simulink model "MICROBOT_1"  (R2015a)
settings: Solver=ode3  StartTime=0.0  StopTime=inf  FixedStep=0.001  RelTol=1e-3
values from neighbouring files (symbols this model uses):
  s = serial('COM4','BaudRate',9600,'DataBits', 8,'Terminator',13)    [start.m]
libraries: mblibv1 x39
settings Model: Creator=anhkh  LastModifiedBy=anhkh
settings SimMechanicsCC: VisOnUpdateDiagram=on  VisDuringSimulation=on

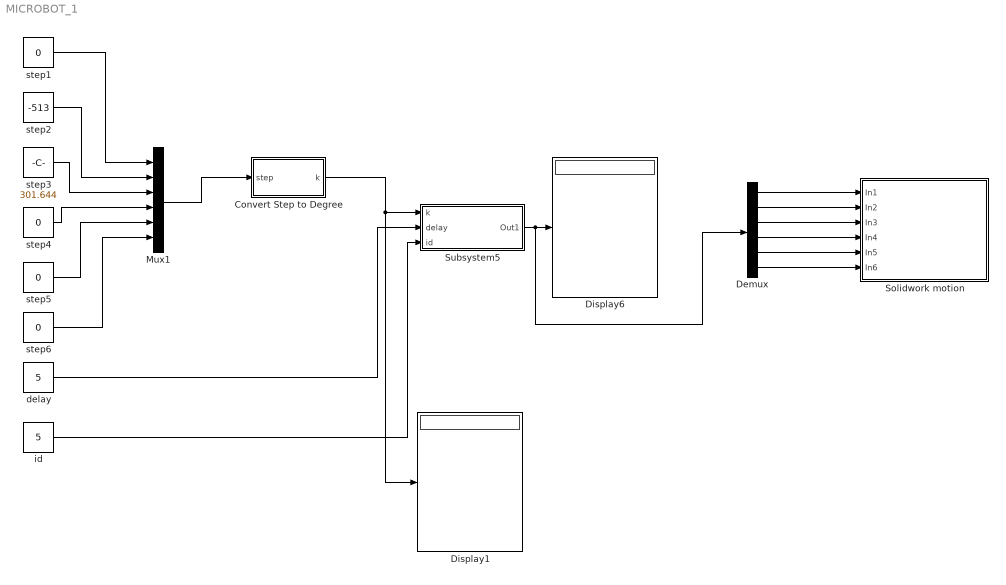
== system MICROBOT_1 ==
  Convert Step to Degree : MATLAB Function  TreatAsAtomicUnit=on
  Demux : Demux  Outputs=6
  Display1 : Display
  Display6 : Display
  Mux1 : Mux  Inputs=6
  Solidwork motion : Subsystem
  Subsystem5 : Subsystem
  delay : Constant  Value=5
  id : Constant  Value=5
  step{1,4..6} (4 alike) : Constant  Value=0
  step2 : Constant  Value=-513
  step3 : Constant  Value=301.644
  wires:
  delay/1 -> Subsystem5/2(delay)
  id/1 -> Subsystem5/3(id)
  Demux/1 -> Solidwork motion/1(In1)
  Demux/2 -> Solidwork motion/2(In2)
  Demux/3 -> Solidwork motion/3(In3)
  Demux/4 -> Solidwork motion/4(In4)
  Demux/5 -> Solidwork motion/5(In5)
  Demux/6 -> Solidwork motion/6(In6)
  Subsystem5/1(Out1) -> Demux/1, Display6/1
  Mux1/1 -> Convert Step to Degree/1(step)
  Convert Step to Degree/1(k) -> Display1/1, Subsystem5/1(k)
  step1/1 -> Mux1/1
  step2/1 -> Mux1/2
  step3/1 -> Mux1/3
  step4/1 -> Mux1/4
  step5/1 -> Mux1/5
  step6/1 -> Mux1/6

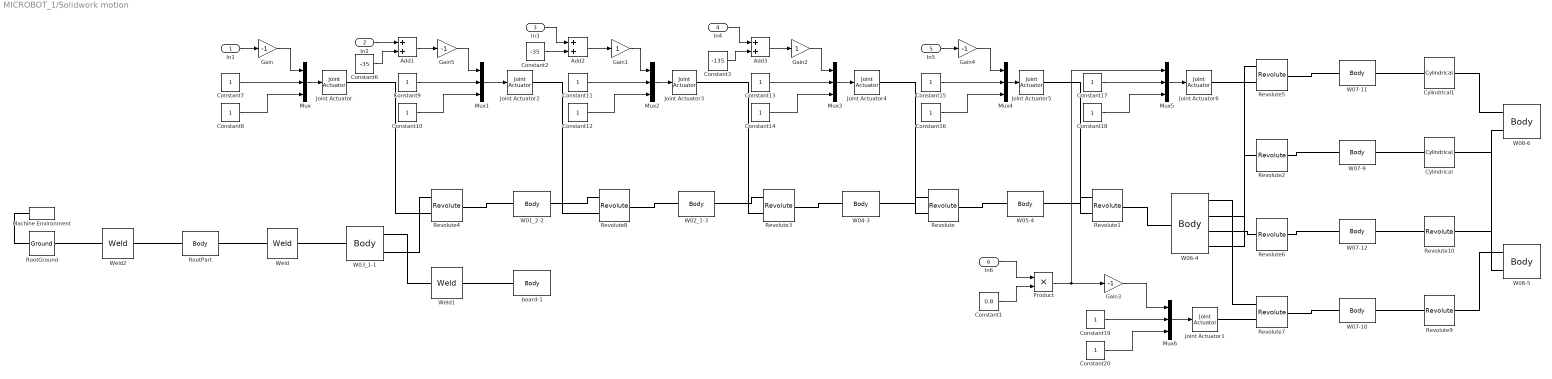
== system MICROBOT_1/Solidwork motion ==
  In1 : Inport
  In2 : Inport  Port=2
  In3 : Inport  Port=3
  In4 : Inport  Port=4
  In5 : Inport  Port=5
  In6 : Inport  Port=6
  Add1 : Sum
  Add2 : Sum
  Add3 : Sum
  Constant1 : Constant  Value=0.8
  Constant{7..20} (14 alike) : Constant
  Constant2 : Constant  Value=-35
  Constant3 : Constant  Value=-135
  Constant6 : Constant  Value=-35
  Cylindrical : mblibv1/Joints/Cylindrical  LConnTagsString=__newl0  RConnTagsString=__newr0  UpdateFromCAD=on  NumSAPorts=0  CutJoint=off  MarkAsCut=off  Primitives=prismatic  PrimitiveProps=P1$WORLD$[0.906308,0,-0.422618]$prismatic#R1$WORLD$[0.906308,0,-0.422618]$revolute  DialogClass=JointBlock  P1Axis=[0.906308,0,-0.422618]  R1Axis=[0.906308,0,-0.422618]
  Cylindrical1 : mblibv1/Joints/Cylindrical  LConnTagsString=__newl0  RConnTagsString=__newr0  UpdateFromCAD=on  NumSAPorts=0  CutJoint=off  MarkAsCut=off  Primitives=prismatic  PrimitiveProps=P1$WORLD$[-0.906308,0,0.422618]$prismatic#R1$WORLD$[0.906308,0,-0.422618]$revolute  DialogClass=JointBlock  P1Axis=[-0.906308,0,0.422618]  R1Axis=[0.906308,0,-0.422618]
  Gain{,3..5} (4 alike) : Gain  Gain=-1
  Gain1 : Gain
  Gain2 : Gain
  Joint Actuator{,1..6} (7 alike) : mblibv1/Sensors &  Actuators/Joint Actuator  UpdateFromCAD=off  PhysicalDomain=Mechanical  PortType=blob  ActuationStyle=Motion  AngleUnits=deg  ArcVelocityUnits=deg/s  ArcAccelerationUnits=deg/s^2  CoordPositionUnits=m  VelocityUnits=m/s  AccelerationUnits=m/s^2  ForceUnits=N  TorqueUnits=N*m  ActiveIO=on  Width=3  DialogClass=MechanicalActuatorBlock  Primitive=R1  ReferenceFrame=Absolute (World)
  Machine Environment : mblibv1/Bodies/Machine Environment  PortType=env  PhysicalDomain=Mechanical  DialogTemplateClass=MECH.MachineEnvironment  SyncWhenCopied=off  Gravity=[0 -9.81 0]  GravityUnits=m/s^2  GravityAsSignal=off  Dimensionality=Auto-detect  AnalysisType=Forward dynamics  LinearAssemblyTolerance=1e-3  LinearAssemblyToleranceUnits=m  AngularAssemblyTolerance=1e-3  AngularAssemblyToleranceUnits=rad  ConstraintSolverType=Stabilizing  ConstraintRelTolerance=1e-4  ConstraintAbsTolerance=1e-4  UseRobustSingularityHandling=off  RedundancyAnalysisToleranceType=Automatically select tolerance  RedundancyAnalysisTolerance=1e-14  StatePerturbationType=Fixed  PerturbationSize=1e-5  VisualizeMachine=on  BodyVisualizationType=Use model default body geometries  BodyColorSelMode=Use model default  DefaultBodyColor=[1 0 0]
  Mux{,1..6} (7 alike) : Mux  Inputs=3
  Product : Product
  Revolute : mblibv1/Joints/Revolute  LConnTagsString=__newl0|SA1  RConnTagsString=__newr0  UpdateFromCAD=on  NumSAPorts=1  CutJoint=off  MarkAsCut=off  Primitives=prismatic  PrimitiveProps=R1$WORLD$[0,1,0]$revolute  DialogClass=JointBlock  R1Axis=[0,1,0]
  Revolute1 : mblibv1/Joints/Revolute  LConnTagsString=__newl0|SA1  RConnTagsString=__newr0  UpdateFromCAD=on  NumSAPorts=1  CutJoint=off  MarkAsCut=off  Primitives=prismatic  PrimitiveProps=R1$WORLD$[0.422618,0,0.906308]$revolute  DialogClass=JointBlock  R1Axis=[0.422618,0,0.906308]
  Revolute10 : mblibv1/Joints/Revolute  LConnTagsString=__newl0  RConnTagsString=__newr0  UpdateFromCAD=on  NumSAPorts=0  CutJoint=off  MarkAsCut=off  Primitives=prismatic  PrimitiveProps=R1$WORLD$[0.906308,0,-0.422618]$revolute  DialogClass=JointBlock  R1Axis=[0.906308,0,-0.422618]
  Revolute2 : mblibv1/Joints/Revolute  LConnTagsString=__newl0  RConnTagsString=__newr0  UpdateFromCAD=on  NumSAPorts=0  CutJoint=off  MarkAsCut=off  Primitives=prismatic  PrimitiveProps=R1$World$[-0.906308,0,0.422618]$revolute  DialogClass=JointBlock  R1Axis=[-0.906308,0,0.422618]
  Revolute3 : mblibv1/Joints/Revolute  LConnTagsString=__newl0|SA1  RConnTagsString=__newr0  UpdateFromCAD=on  NumSAPorts=1  CutJoint=off  MarkAsCut=off  Primitives=prismatic  PrimitiveProps=R1$WORLD$[0,1,0]$revolute  DialogClass=JointBlock  R1Axis=[0,1,0]
  Revolute4 : mblibv1/Joints/Revolute  LConnTagsString=__newl0|SA1  RConnTagsString=__newr0  UpdateFromCAD=on  NumSAPorts=1  CutJoint=off  MarkAsCut=off  Primitives=prismatic  PrimitiveProps=R1$WORLD$[0,0,-1]$revolute  DialogClass=JointBlock  R1Axis=[0,0,-1]
  Revolute5 : mblibv1/Joints/Revolute  LConnTagsString=__newl0|SA1  RConnTagsString=__newr0  UpdateFromCAD=on  NumSAPorts=1  CutJoint=off  MarkAsCut=off  Primitives=prismatic  PrimitiveProps=R1$WORLD$[-0.906308,0,0.422618]$revolute  DialogClass=JointBlock  R1Axis=[-0.906308,0,0.422618]
  Revolute6 : mblibv1/Joints/Revolute  LConnTagsString=__newl0  RConnTagsString=__newr0  UpdateFromCAD=on  NumSAPorts=0  CutJoint=off  MarkAsCut=off  Primitives=prismatic  PrimitiveProps=R1$World$[-0.906308,0,0.422618]$revolute  DialogClass=JointBlock  R1Axis=[-0.906308,0,0.422618]
  Revolute7 : mblibv1/Joints/Revolute  LConnTagsString=__newl0|SA1  RConnTagsString=__newr0  UpdateFromCAD=on  NumSAPorts=1  CutJoint=off  MarkAsCut=off  Primitives=prismatic  PrimitiveProps=R1$WORLD$[-0.906308,0,0.422618]$revolute  DialogClass=JointBlock  R1Axis=[-0.906308,0,0.422618]
  Revolute8 : mblibv1/Joints/Revolute  LConnTagsString=__newl0|SA1  RConnTagsString=__newr0  UpdateFromCAD=on  NumSAPorts=1  CutJoint=off  MarkAsCut=off  Primitives=prismatic  PrimitiveProps=R1$WORLD$[0,-1,0]$revolute  DialogClass=JointBlock  R1Axis=[0,-1,0]
  Revolute9 : mblibv1/Joints/Revolute  LConnTagsString=__newl0  RConnTagsString=__newr0  UpdateFromCAD=on  NumSAPorts=0  CutJoint=off  MarkAsCut=off  Primitives=prismatic  PrimitiveProps=R1$WORLD$[0.906308,0,-0.422618]$revolute  DialogClass=JointBlock  R1Axis=[0.906308,0,-0.422618]
  RootGround : mblibv1/Bodies/Ground  UpdateFromCAD=on  LeftPortType=env  RightPortType=workingframe  PhysicalDomain=Mechanical  DialogClass=GroundBlock  CoordPosition=[-0.110775,0.40847,0.0543535]  CoordPositionUnits=m  StateVectorMgrId=0  MachineId=[1 0]  ShowEnvPort=on  ParameterChecksum=[2042886838, 387347586, 684379528, 2542238582]  TopologyChecksum=[648403851, 3875230276, 106472239, 3042158122]
  RootPart : mblibv1/Bodies/Body  LConnTagsString=CS3  RConnTagsString=CS2  UpdateFromCAD=on  DialogClass=MechanicalBodyBlock  Mass=0  MassUnits=kg  InertiaUnits=kg*m^2  Inertia=[0,0,0;0,0,0;0,0,0]  Shape=Cylinder  ShapeDims=[1 1]  ShapeUnits=m  ShapeUse=false  Density=1  DensityUnits=kg/m^3  DensityUse=false  GraphicsMode=MACHINE_DEFAULT  BodyColorSelMode=MACHINE_DEFAULT  BodyColor=[1;0;0]  AttachedToCS=CS1  CG=Right$CG$[-0.110775 0.40847 0.0543535]$WORLD$WORLD$m$[1 0 0;0 1 0;0 0 1]$3x3 Transform$rad$WORLD$false$none  WorkingFrames=Right$CS1$[0 0 0]$WORLD$WORLD$m$[1 0 0;0 1 0;0 0 1]$3x3 Transform$rad$WORLD$false$none#Right$CS2$[-0.107087 0.143871 0.0371879]$WORLD$WORLD$m$[1 0 0;0 1 0;0 0 1]$3x3 Transform$rad$WORLD$true$none#Left$CS3$[-0.110775 0.40847 0.0543535]$WORLD$WORLD$m$[1 0 0;0 1 0;0 0 1]$3x3 Transform$rad$WORLD$true$none  CGPos=[-0.110775 0.40847 0.0543535]  CGRot=[1 0 0;0 1 0;0 0 1]  CS0Pos=[]  CS0Rot=[]  CS1Pos=[0 0 0]  CS1Rot=[1 0 0;0 1 0;0 0 1]  CS2Pos=[-0.107087 0.143871 0.0371879]  CS2Rot=[1 0 0;0 1 0;0 0 1]  CS3Pos=[-0.110775 0.40847 0.0543535]  CS3Rot=[1 0 0;0 1 0;0 0 1]  CS4Pos=[]  CS4Rot=[]  CS5Pos=[]  CS5Rot=[]  CS6Pos=[]  CS6Rot=[]  CS7Pos=[]  CS7Rot=[]  CS8Pos=[]  CS8Rot=[]  CS9Pos=[]  CS9Rot=[]  CS10Pos=[]  CS10Rot=[]  CS11Pos=[]  CS11Rot=[]  CS12Pos=[]  CS12Rot=[]  CS13Pos=[]  CS13Rot=[]  CS14Pos=[]  CS14Rot=[]  CS15Pos=[]  CS15Rot=[]  CS16Pos=[]  CS16Rot=[]  CS17Pos=[]  CS17Rot=[]  CS18Pos=[]  CS18Rot=[]  CS19Pos=[]  CS19Rot=[]  CS20Pos=[]  CS20Rot=[]
  W01_2-2 : mblibv1/Bodies/Body  LConnTagsString=CS3  RConnTagsString=CS2  UpdateFromCAD=on  DialogClass=MechanicalBodyBlock  Mass=3.41752  MassUnits=kg  InertiaUnits=kg*m^2  Inertia=[0.0156091,-9.74217e-10,-8.96339e-09;-9.74217e-10,0.0136555,0.00112438;-8.96339e-09,0.00112438,0.0159365]  Shape=Cylinder  ShapeDims=[1 1]  ShapeUnits=m  ShapeUse=false  Density=1  DensityUnits=kg/m^3  DensityUse=false  GraphicsMode=GFXFILE  GraphicsFileName=MICROBOT_1 - W01_2-2.STL  BodyColorSelMode=COLORPALETTE  BodyColor=[0.792157;0.819608;0.933333]  AttachedToCS=CS1  CG=Right$CG$[-0.15354 0.221184 0.150881]$WORLD$WORLD$m$[0 1 0;1 0 0;0 0 -1]$3x3 Transform$rad$WORLD$false$none  WorkingFrames=Right$CS1$[-0.157087 0.221184 0.193]$WORLD$WORLD$m$[0 1 0;1 0 0;0 0 -1]$3x3 Transform$rad$WORLD$false$none#Right$CS2$[-0.107087 0.252684 0.243]$WORLD$WORLD$m$[1 0 0;0 1 0;0 0 1]$3x3 Transform$rad$WORLD$true$none#Left$CS3$[-0.107087 0.221184 0.103]$WORLD$WORLD$m$[1 0 0;0 1 0;0 0 1]$3x3 Transform$rad$WORLD$true$none  CGPos=[-0.15354 0.221184 0.150881]  CGRot=[0 1 0;1 0 0;0 0 -1]  CS0Pos=[]  CS0Rot=[]  CS1Pos=[-0.157087 0.221184 0.193]  CS1Rot=[0 1 0;1 0 0;0 0 -1]  CS2Pos=[-0.107087 0.252684 0.243]  CS2Rot=[1 0 0;0 1 0;0 0 1]  CS3Pos=[-0.107087 0.221184 0.103]  CS3Rot=[1 0 0;0 1 0;0 0 1]  CS4Pos=[]  CS4Rot=[]  CS5Pos=[]  CS5Rot=[]  CS6Pos=[]  CS6Rot=[]  CS7Pos=[]  CS7Rot=[]  CS8Pos=[]  CS8Rot=[]  CS9Pos=[]  CS9Rot=[]  CS10Pos=[]  CS10Rot=[]  CS11Pos=[]  CS11Rot=[]  CS12Pos=[]  CS12Rot=[]  CS13Pos=[]  CS13Rot=[]  CS14Pos=[]  CS14Rot=[]  CS15Pos=[]  CS15Rot=[]  CS16Pos=[]  CS16Rot=[]  CS17Pos=[]  CS17Rot=[]  CS18Pos=[]  CS18Rot=[]  CS19Pos=[]  CS19Rot=[]  CS20Pos=[]  CS20Rot=[]
  W02_1-3 : mblibv1/Bodies/Body  LConnTagsString=CS2  RConnTagsString=CS3  UpdateFromCAD=on  DialogClass=MechanicalBodyBlock  Mass=0.137184  MassUnits=kg  InertiaUnits=kg*m^2  Inertia=[0.000250835,-0.000173843,-1.3272e-07;-0.000173843,0.000692155,9.67815e-08;-1.3272e-07,9.67815e-08,0.000724516]  Shape=Cylinder  ShapeDims=[1 1]  ShapeUnits=m  ShapeUse=false  Density=1  DensityUnits=kg/m^3  DensityUse=false  GraphicsMode=GFXFILE  GraphicsFileName=MICROBOT_1 - W02_1-3.STL  BodyColorSelMode=COLORPALETTE  BodyColor=[0.792157;0.819608;0.933333]  AttachedToCS=CS1  CG=Right$CG$[-0.0248881 0.22102 0.249502]$WORLD$WORLD$m$[0.948668 0.316273 0;0 0 -1;-0.316273 0.948668 0]$3x3 Transform$rad$WORLD$false$none  WorkingFrames=Right$CS1$[-0.0240745 0.252684 0.238257]$WORLD$WORLD$m$[0.948668 0.316273 0;0 0 -1;-0.316273 0.948668 0]$3x3 Transform$rad$WORLD$false$none#Left$CS2$[-0.107087 0.252684 0.243]$WORLD$WORLD$m$[1 0 0;0 1 0;0 0 1]$3x3 Transform$rad$WORLD$true$none#Right$CS3$[0.0779125 0.236184 0.243]$WORLD$WORLD$m$[1 0 0;0 1 0;0 0 1]$3x3 Transform$rad$WORLD$true$none  CGPos=[-0.0248881 0.22102 0.249502]  CGRot=[0.948668 0.316273 0;0 0 -1;-0.316273 0.948668 0]  CS0Pos=[]  CS0Rot=[]  CS1Pos=[-0.0240745 0.252684 0.238257]  CS1Rot=[0.948668 0.316273 0;0 0 -1;-0.316273 0.948668 0]  CS2Pos=[-0.107087 0.252684 0.243]  CS2Rot=[1 0 0;0 1 0;0 0 1]  CS3Pos=[0.0779125 0.236184 0.243]  CS3Rot=[1 0 0;0 1 0;0 0 1]  CS4Pos=[]  CS4Rot=[]  CS5Pos=[]  CS5Rot=[]  CS6Pos=[]  CS6Rot=[]  CS7Pos=[]  CS7Rot=[]  CS8Pos=[]  CS8Rot=[]  CS9Pos=[]  CS9Rot=[]  CS10Pos=[]  CS10Rot=[]  CS11Pos=[]  CS11Rot=[]  CS12Pos=[]  CS12Rot=[]  CS13Pos=[]  CS13Rot=[]  CS14Pos=[]  CS14Rot=[]  CS15Pos=[]  CS15Rot=[]  CS16Pos=[]  CS16Rot=[]  CS17Pos=[]  CS17Rot=[]  CS18Pos=[]  CS18Rot=[]  CS19Pos=[]  CS19Rot=[]  CS20Pos=[]  CS20Rot=[]
  W03_1-1 : mblibv1/Bodies/Body  LConnTagsString=CS2  RConnTagsString=CS3|CS4  UpdateFromCAD=on  DialogClass=MechanicalBodyBlock  Mass=3.89994  MassUnits=kg  InertiaUnits=kg*m^2  Inertia=[0.0172249,0,0;0,0.0322437,-3.95609e-05;0,-3.95609e-05,0.0192496]  Shape=Cylinder  ShapeDims=[1 1]  ShapeUnits=m  ShapeUse=false  Density=1  DensityUnits=kg/m^3  DensityUse=false  GraphicsMode=GFXFILE  GraphicsFileName=MICROBOT_1 - W03_1-1.STL  BodyColorSelMode=COLORPALETTE  BodyColor=[0.792157;0.819608;0.933333]  AttachedToCS=CS1  CG=Right$CG$[-0.107087 0.143871 0.0371879]$WORLD$WORLD$m$[-1 0 0;0 0 1;0 1 0]$3x3 Transform$rad$WORLD$false$none  WorkingFrames=Right$CS1$[-0.107087 0.036184 0.04]$WORLD$WORLD$m$[-1 0 0;0 0 1;0 1 0]$3x3 Transform$rad$WORLD$false$none#Left$CS2$[-0.107087 0.143871 0.0371879]$WORLD$WORLD$m$[1 0 0;0 1 0;0 0 1]$3x3 Transform$rad$WORLD$true$none#Right$CS3$[-0.107087 0.036184 -0.02]$WORLD$WORLD$m$[1 0 0;0 1 0;0 0 1]$3x3 Transform$rad$WORLD$true$none#Right$CS4$[-0.107087 0.221184 0.103]$WORLD$WORLD$m$[1 0 0;0 1 0;0 0 1]$3x3 Transform$rad$WORLD$true$none  CGPos=[-0.107087 0.143871 0.0371879]  CGRot=[-1 0 0;0 0 1;0 1 0]  CS0Pos=[]  CS0Rot=[]  CS1Pos=[-0.107087 0.036184 0.04]  CS1Rot=[-1 0 0;0 0 1;0 1 0]  CS2Pos=[-0.107087 0.143871 0.0371879]  CS2Rot=[1 0 0;0 1 0;0 0 1]  CS3Pos=[-0.107087 0.036184 -0.02]  CS3Rot=[1 0 0;0 1 0;0 0 1]  CS4Pos=[-0.107087 0.221184 0.103]  CS4Rot=[1 0 0;0 1 0;0 0 1]  CS5Pos=[]  CS5Rot=[]  CS6Pos=[]  CS6Rot=[]  CS7Pos=[]  CS7Rot=[]  CS8Pos=[]  CS8Rot=[]  CS9Pos=[]  CS9Rot=[]  CS10Pos=[]  CS10Rot=[]  CS11Pos=[]  CS11Rot=[]  CS12Pos=[]  CS12Rot=[]  CS13Pos=[]  CS13Rot=[]  CS14Pos=[]  CS14Rot=[]  CS15Pos=[]  CS15Rot=[]  CS16Pos=[]  CS16Rot=[]  CS17Pos=[]  CS17Rot=[]  CS18Pos=[]  CS18Rot=[]  CS19Pos=[]  CS19Rot=[]  CS20Pos=[]  CS20Rot=[]
  W04-3 : mblibv1/Bodies/Body  LConnTagsString=CS2  RConnTagsString=CS3  UpdateFromCAD=on  DialogClass=MechanicalBodyBlock  Mass=0.028469  MassUnits=kg  InertiaUnits=kg*m^2  Inertia=[0.00010055,-1.1564e-07,2.98034e-07;-1.1564e-07,0.000108696,-6.97188e-07;2.98034e-07,-6.97188e-07,2.10954e-05]  Shape=Cylinder  ShapeDims=[1 1]  ShapeUnits=m  ShapeUse=false  Density=1  DensityUnits=kg/m^3  DensityUse=false  GraphicsMode=GFXFILE  GraphicsFileName=MICROBOT_1 - W04-3.STL  BodyColorSelMode=COLORPALETTE  BodyColor=[0.792157;0.819608;0.933333]  AttachedToCS=CS1  CG=Right$CG$[0.0151194 0.221868 0.199313]$WORLD$WORLD$m$[0 -0.5 0.866025;1 0 0;0 0.866025 0.5]$3x3 Transform$rad$WORLD$false$none  WorkingFrames=Right$CS1$[0.0779125 0.221184 0.243]$WORLD$WORLD$m$[0 -0.5 0.866025;1 0 0;0 0.866025 0.5]$3x3 Transform$rad$WORLD$false$none#Left$CS2$[0.0779125 0.236184 0.243]$WORLD$WORLD$m$[1 0 0;0 1 0;0 0 1]$3x3 Transform$rad$WORLD$true$none#Right$CS3$[-0.0779721 0.247184 0.153]$WORLD$WORLD$m$[1 0 0;0 1 0;0 0 1]$3x3 Transform$rad$WORLD$true$none  CGPos=[0.0151194 0.221868 0.199313]  CGRot=[0 -0.5 0.866025;1 0 0;0 0.866025 0.5]  CS0Pos=[]  CS0Rot=[]  CS1Pos=[0.0779125 0.221184 0.243]  CS1Rot=[0 -0.5 0.866025;1 0 0;0 0.866025 0.5]  CS2Pos=[0.0779125 0.236184 0.243]  CS2Rot=[1 0 0;0 1 0;0 0 1]  CS3Pos=[-0.0779721 0.247184 0.153]  CS3Rot=[1 0 0;0 1 0;0 0 1]  CS4Pos=[]  CS4Rot=[]  CS5Pos=[]  CS5Rot=[]  CS6Pos=[]  CS6Rot=[]  CS7Pos=[]  CS7Rot=[]  CS8Pos=[]  CS8Rot=[]  CS9Pos=[]  CS9Rot=[]  CS10Pos=[]  CS10Rot=[]  CS11Pos=[]  CS11Rot=[]  CS12Pos=[]  CS12Rot=[]  CS13Pos=[]  CS13Rot=[]  CS14Pos=[]  CS14Rot=[]  CS15Pos=[]  CS15Rot=[]  CS16Pos=[]  CS16Rot=[]  CS17Pos=[]  CS17Rot=[]  CS18Pos=[]  CS18Rot=[]  CS19Pos=[]  CS19Rot=[]  CS20Pos=[]  CS20Rot=[]
  W05-4 : mblibv1/Bodies/Body  LConnTagsString=CS2  RConnTagsString=CS3  UpdateFromCAD=on  DialogClass=MechanicalBodyBlock  Mass=0.0114047  MassUnits=kg  InertiaUnits=kg*m^2  Inertia=[7.08852e-07,0,6.72492e-12;0,1.28223e-06,-2.77128e-11;6.72492e-12,-2.77128e-11,1.23052e-06]  Shape=Cylinder  ShapeDims=[1 1]  ShapeUnits=m  ShapeUse=false  Density=1  DensityUnits=kg/m^3  DensityUse=false  GraphicsMode=GFXFILE  GraphicsFileName=MICROBOT_1 - W05-4.STL  BodyColorSelMode=COLORPALETTE  BodyColor=[0.792157;0.819608;0.933333]  AttachedToCS=CS1  CG=Right$CG$[-0.078159 0.221184 0.152599]$WORLD$WORLD$m$[0 -0.422618 -0.906308;1 0 0;0 -0.906308 0.422618]$3x3 Transform$rad$WORLD$false$none  WorkingFrames=Right$CS1$[-0.0779721 0.221184 0.153]$WORLD$WORLD$m$[0 -0.422618 -0.906308;1 0 0;0 -0.906308 0.422618]$3x3 Transform$rad$WORLD$false$none#Left$CS2$[-0.0779721 0.247184 0.153]$WORLD$WORLD$m$[1 0 0;0 1 0;0 0 1]$3x3 Transform$rad$WORLD$true$none#Right$CS3$[-0.0787747 0.221184 0.151279]$WORLD$WORLD$m$[1 0 0;0 1 0;0 0 1]$3x3 Transform$rad$WORLD$true$none  CGPos=[-0.078159 0.221184 0.152599]  CGRot=[0 -0.422618 -0.906308;1 0 0;0 -0.906308 0.422618]  CS0Pos=[]  CS0Rot=[]  CS1Pos=[-0.0779721 0.221184 0.153]  CS1Rot=[0 -0.422618 -0.906308;1 0 0;0 -0.906308 0.422618]  CS2Pos=[-0.0779721 0.247184 0.153]  CS2Rot=[1 0 0;0 1 0;0 0 1]  CS3Pos=[-0.0787747 0.221184 0.151279]  CS3Rot=[1 0 0;0 1 0;0 0 1]  CS4Pos=[]  CS4Rot=[]  CS5Pos=[]  CS5Rot=[]  CS6Pos=[]  CS6Rot=[]  CS7Pos=[]  CS7Rot=[]  CS8Pos=[]  CS8Rot=[]  CS9Pos=[]  CS9Rot=[]  CS10Pos=[]  CS10Rot=[]  CS11Pos=[]  CS11Rot=[]  CS12Pos=[]  CS12Rot=[]  CS13Pos=[]  CS13Rot=[]  CS14Pos=[]  CS14Rot=[]  CS15Pos=[]  CS15Rot=[]  CS16Pos=[]  CS16Rot=[]  CS17Pos=[]  CS17Rot=[]  CS18Pos=[]  CS18Rot=[]  CS19Pos=[]  CS19Rot=[]  CS20Pos=[]  CS20Rot=[]
  W06-4 : mblibv1/Bodies/Body  LConnTagsString=CS3  RConnTagsString=CS2|CS4|CS5|CS6  UpdateFromCAD=on  DialogClass=MechanicalBodyBlock  Mass=0.00360366  MassUnits=kg  InertiaUnits=kg*m^2  Inertia=[3.16611e-07,4.38162e-09,0;4.38162e-09,1.36274e-06,0;0,0,1.31379e-06]  Shape=Cylinder  ShapeDims=[1 1]  ShapeUnits=m  ShapeUse=false  Density=1  DensityUnits=kg/m^3  DensityUse=false  GraphicsMode=GFXFILE  GraphicsFileName=MICROBOT_1 - W06-4.STL  BodyColorSelMode=COLORPALETTE  BodyColor=[0;0;0]  AttachedToCS=CS1  CG=Right$CG$[-0.0692621 0.221314 0.171679]$WORLD$WORLD$m$[0 -0.422618 -0.906308;1 0 0;0 -0.906308 0.422618]$3x3 Transform$rad$WORLD$false$none  WorkingFrames=Right$CS1$[-0.0673339 0.221184 0.175814]$WORLD$WORLD$m$[0 -0.422618 -0.906308;1 0 0;0 -0.906308 0.422618]$3x3 Transform$rad$WORLD$false$none#Right$CS2$[-0.0754296 0.199184 0.177382]$WORLD$WORLD$m$[1 0 0;0 1 0;0 0 1]$3x3 Transform$rad$WORLD$true$none#Left$CS3$[-0.0787747 0.221184 0.151279]$WORLD$WORLD$m$[1 0 0;0 1 0;0 0 1]$3x3 Transform$rad$WORLD$true$none#Right$CS4$[-0.0754296 0.243184 0.177382]$WORLD$WORLD$m$[1 0 0;0 1 0;0 0 1]$3x3 Transform$rad$WORLD$true$none#Right$CS5$[-0.0754296 0.251184 0.177382]$WORLD$WORLD$m$[1 0 0;0 1 0;0 0 1]$3x3 Transform$rad$WORLD$true$none#Right$CS6$[-0.0754296 0.191184 0.177382]$WORLD$WORLD$m$[1 0 0;0 1 0;0 0 1]$3x3 Transform$rad$WORLD$true$none  CGPos=[-0.0692621 0.221314 0.171679]  CGRot=[0 -0.422618 -0.906308;1 0 0;0 -0.906308 0.422618]  CS0Pos=[]  CS0Rot=[]  CS1Pos=[-0.0673339 0.221184 0.175814]  CS1Rot=[0 -0.422618 -0.906308;1 0 0;0 -0.906308 0.422618]  CS2Pos=[-0.0754296 0.199184 0.177382]  CS2Rot=[1 0 0;0 1 0;0 0 1]  CS3Pos=[-0.0787747 0.221184 0.151279]  CS3Rot=[1 0 0;0 1 0;0 0 1]  CS4Pos=[-0.0754296 0.243184 0.177382]  CS4Rot=[1 0 0;0 1 0;0 0 1]  CS5Pos=[-0.0754296 0.251184 0.177382]  CS5Rot=[1 0 0;0 1 0;0 0 1]  CS6Pos=[-0.0754296 0.191184 0.177382]  CS6Rot=[1 0 0;0 1 0;0 0 1]  CS7Pos=[]  CS7Rot=[]  CS8Pos=[]  CS8Rot=[]  CS9Pos=[]  CS9Rot=[]  CS10Pos=[]  CS10Rot=[]  CS11Pos=[]  CS11Rot=[]  CS12Pos=[]  CS12Rot=[]  CS13Pos=[]  CS13Rot=[]  CS14Pos=[]  CS14Rot=[]  CS15Pos=[]  CS15Rot=[]  CS16Pos=[]  CS16Rot=[]  CS17Pos=[]  CS17Rot=[]  CS18Pos=[]  CS18Rot=[]  CS19Pos=[]  CS19Rot=[]  CS20Pos=[]  CS20Rot=[]
  W07-10 : mblibv1/Bodies/Body  LConnTagsString=CS3  RConnTagsString=CS2  UpdateFromCAD=on  DialogClass=MechanicalBodyBlock  Mass=0.00554345  MassUnits=kg  InertiaUnits=kg*m^2  Inertia=[1.25755e-06,0,0;0,1.41119e-07,0;0,0,1.16215e-06]  Shape=Cylinder  ShapeDims=[1 1]  ShapeUnits=m  ShapeUse=false  Density=1  DensityUnits=kg/m^3  DensityUse=false  GraphicsMode=GFXFILE  GraphicsFileName=MICROBOT_1 - W07-10.STL  BodyColorSelMode=COLORPALETTE  BodyColor=[0;0;0]  AttachedToCS=CS1  CG=Right$CG$[-0.0597931 0.208684 0.191985]$WORLD$WORLD$m$[-0.182494 -0.381185 -0.906308;0.901961 -0.431818 0;-0.39136 -0.817454 0.422618]$3x3 Transform$rad$WORLD$false$none  WorkingFrames=Right$CS1$[-0.0543552 0.208684 0.189449]$WORLD$WORLD$m$[-0.182494 -0.381185 -0.906308;0.901961 -0.431818 0;-0.39136 -0.817454 0.422618]$3x3 Transform$rad$WORLD$false$none#Right$CS2$[-0.0586575 0.218184 0.21335]$WORLD$WORLD$m$[1 0 0;0 1 0;0 0 1]$3x3 Transform$rad$WORLD$true$none#Left$CS3$[-0.0754296 0.199184 0.177382]$WORLD$WORLD$m$[1 0 0;0 1 0;0 0 1]$3x3 Transform$rad$WORLD$true$none  CGPos=[-0.0597931 0.208684 0.191985]  CGRot=[-0.182494 -0.381185 -0.906308;0.901961 -0.431818 0;-0.39136 -0.817454 0.422618]  CS0Pos=[]  CS0Rot=[]  CS1Pos=[-0.0543552 0.208684 0.189449]  CS1Rot=[-0.182494 -0.381185 -0.906308;0.901961 -0.431818 0;-0.39136 -0.817454 0.422618]  CS2Pos=[-0.0586575 0.218184 0.21335]  CS2Rot=[1 0 0;0 1 0;0 0 1]  CS3Pos=[-0.0754296 0.199184 0.177382]  CS3Rot=[1 0 0;0 1 0;0 0 1]  CS4Pos=[]  CS4Rot=[]  CS5Pos=[]  CS5Rot=[]  CS6Pos=[]  CS6Rot=[]  CS7Pos=[]  CS7Rot=[]  CS8Pos=[]  CS8Rot=[]  CS9Pos=[]  CS9Rot=[]  CS10Pos=[]  CS10Rot=[]  CS11Pos=[]  CS11Rot=[]  CS12Pos=[]  CS12Rot=[]  CS13Pos=[]  CS13Rot=[]  CS14Pos=[]  CS14Rot=[]  CS15Pos=[]  CS15Rot=[]  CS16Pos=[]  CS16Rot=[]  CS17Pos=[]  CS17Rot=[]  CS18Pos=[]  CS18Rot=[]  CS19Pos=[]  CS19Rot=[]  CS20Pos=[]  CS20Rot=[]
  W07-11 : mblibv1/Bodies/Body  LConnTagsString=CS3  RConnTagsString=CS2  UpdateFromCAD=on  DialogClass=MechanicalBodyBlock  Mass=0.00554345  MassUnits=kg  InertiaUnits=kg*m^2  Inertia=[1.25755e-06,0,0;0,1.41119e-07,0;0,0,1.16215e-06]  Shape=Cylinder  ShapeDims=[1 1]  ShapeUnits=m  ShapeUse=false  Density=1  DensityUnits=kg/m^3  DensityUse=false  GraphicsMode=GFXFILE  GraphicsFileName=MICROBOT_1 - W07-11.STL  BodyColorSelMode=COLORPALETTE  BodyColor=[0;0;0]  AttachedToCS=CS1  CG=Right$CG$[-0.0597931 0.233684 0.191985]$WORLD$WORLD$m$[0.182494 -0.381185 -0.906308;0.901961 0.431818 0;0.39136 -0.817454 0.422618]$3x3 Transform$rad$WORLD$false$none  WorkingFrames=Right$CS1$[-0.0543552 0.233684 0.189449]$WORLD$WORLD$m$[0.182494 -0.381185 -0.906308;0.901961 0.431818 0;0.39136 -0.817454 0.422618]$3x3 Transform$rad$WORLD$false$none#Right$CS2$[-0.0586575 0.224184 0.21335]$WORLD$WORLD$m$[1 0 0;0 1 0;0 0 1]$3x3 Transform$rad$WORLD$true$none#Left$CS3$[-0.0754296 0.243184 0.177382]$WORLD$WORLD$m$[1 0 0;0 1 0;0 0 1]$3x3 Transform$rad$WORLD$true$none  CGPos=[-0.0597931 0.233684 0.191985]  CGRot=[0.182494 -0.381185 -0.906308;0.901961 0.431818 0;0.39136 -0.817454 0.422618]  CS0Pos=[]  CS0Rot=[]  CS1Pos=[-0.0543552 0.233684 0.189449]  CS1Rot=[0.182494 -0.381185 -0.906308;0.901961 0.431818 0;0.39136 -0.817454 0.422618]  CS2Pos=[-0.0586575 0.224184 0.21335]  CS2Rot=[1 0 0;0 1 0;0 0 1]  CS3Pos=[-0.0754296 0.243184 0.177382]  CS3Rot=[1 0 0;0 1 0;0 0 1]  CS4Pos=[]  CS4Rot=[]  CS5Pos=[]  CS5Rot=[]  CS6Pos=[]  CS6Rot=[]  CS7Pos=[]  CS7Rot=[]  CS8Pos=[]  CS8Rot=[]  CS9Pos=[]  CS9Rot=[]  CS10Pos=[]  CS10Rot=[]  CS11Pos=[]  CS11Rot=[]  CS12Pos=[]  CS12Rot=[]  CS13Pos=[]  CS13Rot=[]  CS14Pos=[]  CS14Rot=[]  CS15Pos=[]  CS15Rot=[]  CS16Pos=[]  CS16Rot=[]  CS17Pos=[]  CS17Rot=[]  CS18Pos=[]  CS18Rot=[]  CS19Pos=[]  CS19Rot=[]  CS20Pos=[]  CS20Rot=[]
  W07-12 : mblibv1/Bodies/Body  LConnTagsString=CS3  RConnTagsString=CS2  UpdateFromCAD=on  DialogClass=MechanicalBodyBlock  Mass=0.00554345  MassUnits=kg  InertiaUnits=kg*m^2  Inertia=[1.25755e-06,0,0;0,1.41119e-07,0;0,0,1.16215e-06]  Shape=Cylinder  ShapeDims=[1 1]  ShapeUnits=m  ShapeUse=false  Density=1  DensityUnits=kg/m^3  DensityUse=false  GraphicsMode=GFXFILE  GraphicsFileName=MICROBOT_1 - W07-12.STL  BodyColorSelMode=COLORPALETTE  BodyColor=[0;0;0]  AttachedToCS=CS1  CG=Right$CG$[-0.0597931 0.241684 0.191985]$WORLD$WORLD$m$[0.182494 -0.381185 -0.906308;0.901961 0.431818 0;0.39136 -0.817454 0.422618]$3x3 Transform$rad$WORLD$false$none  WorkingFrames=Right$CS1$[-0.0543552 0.241684 0.189449]$WORLD$WORLD$m$[0.182494 -0.381185 -0.906308;0.901961 0.431818 0;0.39136 -0.817454 0.422618]$3x3 Transform$rad$WORLD$false$none#Right$CS2$[-0.0586575 0.232184 0.21335]$WORLD$WORLD$m$[1 0 0;0 1 0;0 0 1]$3x3 Transform$rad$WORLD$true$none#Left$CS3$[-0.0754296 0.251184 0.177382]$WORLD$WORLD$m$[1 0 0;0 1 0;0 0 1]$3x3 Transform$rad$WORLD$true$none  CGPos=[-0.0597931 0.241684 0.191985]  CGRot=[0.182494 -0.381185 -0.906308;0.901961 0.431818 0;0.39136 -0.817454 0.422618]  CS0Pos=[]  CS0Rot=[]  CS1Pos=[-0.0543552 0.241684 0.189449]  CS1Rot=[0.182494 -0.381185 -0.906308;0.901961 0.431818 0;0.39136 -0.817454 0.422618]  CS2Pos=[-0.0586575 0.232184 0.21335]  CS2Rot=[1 0 0;0 1 0;0 0 1]  CS3Pos=[-0.0754296 0.251184 0.177382]  CS3Rot=[1 0 0;0 1 0;0 0 1]  CS4Pos=[]  CS4Rot=[]  CS5Pos=[]  CS5Rot=[]  CS6Pos=[]  CS6Rot=[]  CS7Pos=[]  CS7Rot=[]  CS8Pos=[]  CS8Rot=[]  CS9Pos=[]  CS9Rot=[]  CS10Pos=[]  CS10Rot=[]  CS11Pos=[]  CS11Rot=[]  CS12Pos=[]  CS12Rot=[]  CS13Pos=[]  CS13Rot=[]  CS14Pos=[]  CS14Rot=[]  CS15Pos=[]  CS15Rot=[]  CS16Pos=[]  CS16Rot=[]  CS17Pos=[]  CS17Rot=[]  CS18Pos=[]  CS18Rot=[]  CS19Pos=[]  CS19Rot=[]  CS20Pos=[]  CS20Rot=[]
  W07-9 : mblibv1/Bodies/Body  LConnTagsString=CS3  RConnTagsString=CS2  UpdateFromCAD=on  DialogClass=MechanicalBodyBlock  Mass=0.00554345  MassUnits=kg  InertiaUnits=kg*m^2  Inertia=[1.25755e-06,0,0;0,1.41119e-07,0;0,0,1.16215e-06]  Shape=Cylinder  ShapeDims=[1 1]  ShapeUnits=m  ShapeUse=false  Density=1  DensityUnits=kg/m^3  DensityUse=false  GraphicsMode=GFXFILE  GraphicsFileName=MICROBOT_1 - W07-9.STL  BodyColorSelMode=COLORPALETTE  BodyColor=[0;0;0]  AttachedToCS=CS1  CG=Right$CG$[-0.0597931 0.200684 0.191985]$WORLD$WORLD$m$[-0.182494 -0.381185 -0.906308;0.901961 -0.431818 0;-0.39136 -0.817454 0.422618]$3x3 Transform$rad$WORLD$false$none  WorkingFrames=Right$CS1$[-0.0543552 0.200684 0.189449]$WORLD$WORLD$m$[-0.182494 -0.381185 -0.906308;0.901961 -0.431818 0;-0.39136 -0.817454 0.422618]$3x3 Transform$rad$WORLD$false$none#Right$CS2$[-0.0586575 0.210184 0.21335]$WORLD$WORLD$m$[1 0 0;0 1 0;0 0 1]$3x3 Transform$rad$WORLD$true$none#Left$CS3$[-0.0754296 0.191184 0.177382]$WORLD$WORLD$m$[1 0 0;0 1 0;0 0 1]$3x3 Transform$rad$WORLD$true$none  CGPos=[-0.0597931 0.200684 0.191985]  CGRot=[-0.182494 -0.381185 -0.906308;0.901961 -0.431818 0;-0.39136 -0.817454 0.422618]  CS0Pos=[]  CS0Rot=[]  CS1Pos=[-0.0543552 0.200684 0.189449]  CS1Rot=[-0.182494 -0.381185 -0.906308;0.901961 -0.431818 0;-0.39136 -0.817454 0.422618]  CS2Pos=[-0.0586575 0.210184 0.21335]  CS2Rot=[1 0 0;0 1 0;0 0 1]  CS3Pos=[-0.0754296 0.191184 0.177382]  CS3Rot=[1 0 0;0 1 0;0 0 1]  CS4Pos=[]  CS4Rot=[]  CS5Pos=[]  CS5Rot=[]  CS6Pos=[]  CS6Rot=[]  CS7Pos=[]  CS7Rot=[]  CS8Pos=[]  CS8Rot=[]  CS9Pos=[]  CS9Rot=[]  CS10Pos=[]  CS10Rot=[]  CS11Pos=[]  CS11Rot=[]  CS12Pos=[]  CS12Rot=[]  CS13Pos=[]  CS13Rot=[]  CS14Pos=[]  CS14Rot=[]  CS15Pos=[]  CS15Rot=[]  CS16Pos=[]  CS16Rot=[]  CS17Pos=[]  CS17Rot=[]  CS18Pos=[]  CS18Rot=[]  CS19Pos=[]  CS19Rot=[]  CS20Pos=[]  CS20Rot=[]
  W08-5 : mblibv1/Bodies/Body  LConnTagsString=CS2|CS3  UpdateFromCAD=on  DialogClass=MechanicalBodyBlock  Mass=0.000736673  MassUnits=kg  InertiaUnits=kg*m^2  Inertia=[7.2718e-08,9.77805e-09,0;9.77805e-09,5.45667e-08,0;0,0,4.04479e-08]  Shape=Cylinder  ShapeDims=[1 1]  ShapeUnits=m  ShapeUse=false  Density=1  DensityUnits=kg/m^3  DensityUse=false  GraphicsMode=GFXFILE  GraphicsFileName=MICROBOT_1 - W08-5.STL  BodyColorSelMode=COLORPALETTE  BodyColor=[0;0;0]  AttachedToCS=CS1  CG=Right$CG$[-0.0473398 0.217519 0.217508]$WORLD$WORLD$m$[0 -0.422618 -0.906308;1 0 0;0 -0.906308 0.422618]$3x3 Transform$rad$WORLD$false$none  WorkingFrames=Right$CS1$[-0.0522217 0.221184 0.207039]$WORLD$WORLD$m$[0 -0.422618 -0.906308;1 0 0;0 -0.906308 0.422618]$3x3 Transform$rad$WORLD$false$none#Left$CS2$[-0.0586575 0.218184 0.21335]$WORLD$WORLD$m$[1 0 0;0 1 0;0 0 1]$3x3 Transform$rad$WORLD$true$none#Left$CS3$[-0.0586575 0.210184 0.21335]$WORLD$WORLD$m$[1 0 0;0 1 0;0 0 1]$3x3 Transform$rad$WORLD$true$none  CGPos=[-0.0473398 0.217519 0.217508]  CGRot=[0 -0.422618 -0.906308;1 0 0;0 -0.906308 0.422618]  CS0Pos=[]  CS0Rot=[]  CS1Pos=[-0.0522217 0.221184 0.207039]  CS1Rot=[0 -0.422618 -0.906308;1 0 0;0 -0.906308 0.422618]  CS2Pos=[-0.0586575 0.218184 0.21335]  CS2Rot=[1 0 0;0 1 0;0 0 1]  CS3Pos=[-0.0586575 0.210184 0.21335]  CS3Rot=[1 0 0;0 1 0;0 0 1]  CS4Pos=[]  CS4Rot=[]  CS5Pos=[]  CS5Rot=[]  CS6Pos=[]  CS6Rot=[]  CS7Pos=[]  CS7Rot=[]  CS8Pos=[]  CS8Rot=[]  CS9Pos=[]  CS9Rot=[]  CS10Pos=[]  CS10Rot=[]  CS11Pos=[]  CS11Rot=[]  CS12Pos=[]  CS12Rot=[]  CS13Pos=[]  CS13Rot=[]  CS14Pos=[]  CS14Rot=[]  CS15Pos=[]  CS15Rot=[]  CS16Pos=[]  CS16Rot=[]  CS17Pos=[]  CS17Rot=[]  CS18Pos=[]  CS18Rot=[]  CS19Pos=[]  CS19Rot=[]  CS20Pos=[]  CS20Rot=[]
  W08-6 : mblibv1/Bodies/Body  LConnTagsString=CS2|CS3  UpdateFromCAD=on  DialogClass=MechanicalBodyBlock  Mass=0.000736673  MassUnits=kg  InertiaUnits=kg*m^2  Inertia=[7.2718e-08,9.77805e-09,0;9.77805e-09,5.45667e-08,0;0,0,4.04479e-08]  Shape=Cylinder  ShapeDims=[1 1]  ShapeUnits=m  ShapeUse=false  Density=1  DensityUnits=kg/m^3  DensityUse=false  GraphicsMode=GFXFILE  GraphicsFileName=MICROBOT_1 - W08-6.STL  BodyColorSelMode=COLORPALETTE  BodyColor=[0;0;0]  AttachedToCS=CS1  CG=Right$CG$[-0.0473398 0.224849 0.217508]$WORLD$WORLD$m$[0 -0.422618 0.906308;-1 0 0;0 -0.906308 -0.422618]$3x3 Transform$rad$WORLD$false$none  WorkingFrames=Right$CS1$[-0.0522217 0.221184 0.207039]$WORLD$WORLD$m$[0 -0.422618 0.906308;-1 0 0;0 -0.906308 -0.422618]$3x3 Transform$rad$WORLD$false$none#Left$CS2$[-0.0586575 0.224184 0.21335]$WORLD$WORLD$m$[1 0 0;0 1 0;0 0 1]$3x3 Transform$rad$WORLD$true$none#Left$CS3$[-0.0586575 0.232184 0.21335]$WORLD$WORLD$m$[1 0 0;0 1 0;0 0 1]$3x3 Transform$rad$WORLD$true$none  CGPos=[-0.0473398 0.224849 0.217508]  CGRot=[0 -0.422618 0.906308;-1 0 0;0 -0.906308 -0.422618]  CS0Pos=[]  CS0Rot=[]  CS1Pos=[-0.0522217 0.221184 0.207039]  CS1Rot=[0 -0.422618 0.906308;-1 0 0;0 -0.906308 -0.422618]  CS2Pos=[-0.0586575 0.224184 0.21335]  CS2Rot=[1 0 0;0 1 0;0 0 1]  CS3Pos=[-0.0586575 0.232184 0.21335]  CS3Rot=[1 0 0;0 1 0;0 0 1]  CS4Pos=[]  CS4Rot=[]  CS5Pos=[]  CS5Rot=[]  CS6Pos=[]  CS6Rot=[]  CS7Pos=[]  CS7Rot=[]  CS8Pos=[]  CS8Rot=[]  CS9Pos=[]  CS9Rot=[]  CS10Pos=[]  CS10Rot=[]  CS11Pos=[]  CS11Rot=[]  CS12Pos=[]  CS12Rot=[]  CS13Pos=[]  CS13Rot=[]  CS14Pos=[]  CS14Rot=[]  CS15Pos=[]  CS15Rot=[]  CS16Pos=[]  CS16Rot=[]  CS17Pos=[]  CS17Rot=[]  CS18Pos=[]  CS18Rot=[]  CS19Pos=[]  CS19Rot=[]  CS20Pos=[]  CS20Rot=[]
  Weld : mblibv1/Joints/Weld  LConnTagsString=__newl0  RConnTagsString=__newr0  UpdateFromCAD=on  NumSAPorts=0  CutJoint=off  MarkAsCut=off  Primitives=weld  PrimitiveProps=W$WORLD$[0.57735,0.57735,0.57735]$weld  DialogClass=JointBlock  WAxis=[0.57735,0.57735,0.57735]
  Weld1 : mblibv1/Joints/Weld  LConnTagsString=__newl0  RConnTagsString=__newr0  UpdateFromCAD=on  NumSAPorts=0  CutJoint=off  MarkAsCut=off  Primitives=weld  PrimitiveProps=W$WORLD$[0.57735,0.57735,0.57735]$weld  DialogClass=JointBlock  WAxis=[0.57735,0.57735,0.57735]
  Weld2 : mblibv1/Joints/Weld  LConnTagsString=__newl0  RConnTagsString=__newr0  UpdateFromCAD=on  NumSAPorts=0  CutJoint=off  MarkAsCut=off  Primitives=weld  PrimitiveProps=W$WORLD$[0.57735,0.57735,0.57735]$weld  DialogClass=JointBlock  WAxis=[0.57735,0.57735,0.57735]
  board-1 : mblibv1/Bodies/Body  LConnTagsString=CS2  UpdateFromCAD=on  DialogClass=MechanicalBodyBlock  Mass=16.6499  MassUnits=kg  InertiaUnits=kg*m^2  Inertia=[0.354681,0.000443934,-0.000371852;0.000443934,0.564949,0.0503728;-0.000371852,0.0503728,0.428805]  Shape=Cylinder  ShapeDims=[1 1]  ShapeUnits=m  ShapeUse=false  Density=1  DensityUnits=kg/m^3  DensityUse=false  GraphicsMode=GFXFILE  GraphicsFileName=MICROBOT_1 - board-1.STL  BodyColorSelMode=COLORPALETTE  BodyColor=[0.792157;0.819608;0.933333]  AttachedToCS=CS1  CG=Right$CG$[-0.103889 0.511188 0.036415]$WORLD$WORLD$m$[1 0 0;0 0 -1;0 1 0]$3x3 Transform$rad$WORLD$false$none  WorkingFrames=Right$CS1$[-0.103779 0.498684 -0.02]$WORLD$WORLD$m$[1 0 0;0 0 -1;0 1 0]$3x3 Transform$rad$WORLD$false$none#Left$CS2$[-0.107087 0.036184 -0.02]$WORLD$WORLD$m$[1 0 0;0 1 0;0 0 1]$3x3 Transform$rad$WORLD$true$none  CGPos=[-0.103889 0.511188 0.036415]  CGRot=[1 0 0;0 0 -1;0 1 0]  CS0Pos=[]  CS0Rot=[]  CS1Pos=[-0.103779 0.498684 -0.02]  CS1Rot=[1 0 0;0 0 -1;0 1 0]  CS2Pos=[-0.107087 0.036184 -0.02]  CS2Rot=[1 0 0;0 1 0;0 0 1]  CS3Pos=[]  CS3Rot=[]  CS4Pos=[]  CS4Rot=[]  CS5Pos=[]  CS5Rot=[]  CS6Pos=[]  CS6Rot=[]  CS7Pos=[]  CS7Rot=[]  CS8Pos=[]  CS8Rot=[]  CS9Pos=[]  CS9Rot=[]  CS10Pos=[]  CS10Rot=[]  CS11Pos=[]  CS11Rot=[]  CS12Pos=[]  CS12Rot=[]  CS13Pos=[]  CS13Rot=[]  CS14Pos=[]  CS14Rot=[]  CS15Pos=[]  CS15Rot=[]  CS16Pos=[]  CS16Rot=[]  CS17Pos=[]  CS17Rot=[]  CS18Pos=[]  CS18Rot=[]  CS19Pos=[]  CS19Rot=[]  CS20Pos=[]  CS20Rot=[]
  wires:
  Mux/1 -> Joint Actuator/1
  Constant7/1 -> Mux/2
  Constant8/1 -> Mux/3
  Mux1/1 -> Joint Actuator2/1
  Constant9/1 -> Mux1/2
  Constant10/1 -> Mux1/3
  Mux2/1 -> Joint Actuator3/1
  Constant11/1 -> Mux2/2
  Constant12/1 -> Mux2/3
  Mux3/1 -> Joint Actuator4/1
  Constant13/1 -> Mux3/2
  Constant14/1 -> Mux3/3
  Mux4/1 -> Joint Actuator5/1
  Constant15/1 -> Mux4/2
  Constant16/1 -> Mux4/3
  Mux5/1 -> Joint Actuator6/1
  Constant17/1 -> Mux5/2
  Constant18/1 -> Mux5/3
  Mux6/1 -> Joint Actuator1/1
  Constant19/1 -> Mux6/2
  Constant20/1 -> Mux6/3
  Gain/1 -> Mux/1
  In1/1 -> Gain/1
  Add2/1 -> Gain1/1
  Gain1/1 -> Mux2/1
  Add3/1 -> Gain2/1
  Gain2/1 -> Mux3/1
  Gain3/1 -> Mux6/1
  Constant6/1 -> Add1/2
  In2/1 -> Add1/1
  Constant2/1 -> Add2/2
  In3/1 -> Add2/1
  Constant3/1 -> Add3/2
  In4/1 -> Add3/1
  Product/1 -> Mux5/1, Gain3/1
  In6/1 -> Product/1
  Constant1/1 -> Product/2
  In5/1 -> Gain4/1
  Gain4/1 -> Mux4/1
  Add1/1 -> Gain5/1
  Gain5/1 -> Mux1/1
  connections:
  Joint Actuator/RConn1 -- Revolute4/LConn2
  Joint Actuator6/RConn1 -- Revolute5/LConn2
  RootGround/LConn1 -- Machine Environment/RConn1
  Joint Actuator4/RConn1 -- Revolute/LConn2
  Revolute7/LConn2 -- Joint Actuator1/RConn1
  Joint Actuator5/RConn1 -- Revolute1/LConn2
  W04-3/RConn1 -- Revolute/LConn1
  Revolute5/RConn1 -- W07-11/LConn1
  Revolute8/LConn2 -- Joint Actuator2/RConn1
  Joint Actuator3/RConn1 -- Revolute3/LConn2
  W02_1-3/RConn1 -- Revolute3/LConn1
  W07-10/RConn1 -- Revolute9/LConn1
  W07-11/RConn1 -- Cylindrical1/LConn1
  Weld/RConn1 -- W03_1-1/LConn1
  RootPart/RConn1 -- Weld/LConn1
  Revolute/RConn1 -- W05-4/LConn1
  W01_2-2/RConn1 -- Revolute8/LConn1
  Revolute7/RConn1 -- W07-10/LConn1
  Revolute4/RConn1 -- W01_2-2/LConn1
  W07-9/RConn1 -- Cylindrical/LConn1
  Revolute3/RConn1 -- W04-3/LConn1
  W06-4/RConn2 -- Revolute5/LConn1
  W03_1-1/RConn1 -- Weld1/LConn1
  Weld1/RConn1 -- board-1/LConn1
  Cylindrical1/RConn1 -- W08-6/LConn1
  Revolute8/RConn1 -- W02_1-3/LConn1
  Cylindrical/RConn1 -- W08-5/LConn2
  W03_1-1/RConn2 -- Revolute4/LConn1
  W06-4/RConn1 -- Revolute7/LConn1
  Revolute1/RConn1 -- W06-4/LConn1
  W05-4/RConn1 -- Revolute1/LConn1
  Revolute9/RConn1 -- W08-5/LConn1
  W06-4/RConn4 -- Revolute2/LConn1
  W07-12/RConn1 -- Revolute10/LConn1
  Revolute6/RConn1 -- W07-12/LConn1
  Revolute10/RConn1 -- W08-6/LConn2
  W06-4/RConn3 -- Revolute6/LConn1
  RootGround/RConn1 -- Weld2/LConn1
  Revolute2/RConn1 -- W07-9/LConn1
  Weld2/RConn1 -- RootPart/LConn1

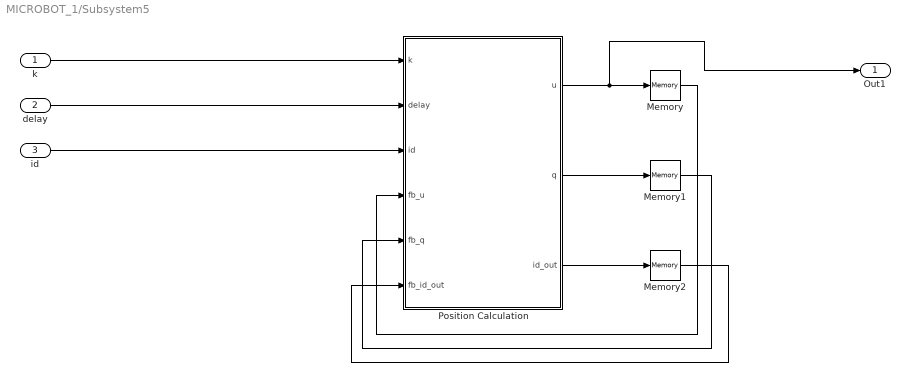
== system MICROBOT_1/Subsystem5 ==
  k : Inport
  delay : Inport  Port=2
  id : Inport  Port=3
  Memory : Memory  X0=[0, 0 ,0, 0, 0, 0]
  Memory1 : Memory  X0=[0, 0 ,0, 0, 0, 0]
  Memory2 : Memory
  "Position Calculation " : MATLAB Function  TreatAsAtomicUnit=on
  Out1 : Outport
  wires:
  k/1 -> "Position Calculation "/1(k)
  delay/1 -> "Position Calculation "/2(delay)
  "Position Calculation "/1(u) -> Out1/1, Memory/1
  "Position Calculation "/2(q) -> Memory1/1
  "Position Calculation "/3(id_out) -> Memory2/1
  Memory/1 -> "Position Calculation "/4(fb_u)
  Memory1/1 -> "Position Calculation "/5(fb_q)
  id/1 -> "Position Calculation "/3(id)
  Memory2/1 -> "Position Calculation "/6(fb_id_out)

== matlab function MICROBOT_1/Convert Step to Degree ==
  data: k output; step input
function k = fcn(step)
%#codegen  
 result = zeros(1,6);
 result(1) = step(1) / 19.64;
 result(2) = step(2) / 19.64;
 result(3) = step(3) / 11.55;
 result(4) = step(4) / 4.27;
 result(5) = step(5) / 4.27;
 result(6) = step(6) / 14.33;
k = result;

== matlab function MICROBOT_1/Subsystem5/Position Calculation  ==
  data: u output; k input; q output; delay input; id input; fb_u input; fb_q input; id_out output; fb_id_out input
function [u, q, id_out] = fcn(k, delay, id, fb_u, fb_q, fb_id_out)
%#codegen  
    
    temp1 = fb_u;
    temp2 = fb_q;
    ts = 0.03;
    ns = delay / ts;
    k_tmp = k;
%     if k_tmp(3) == k_tmp(6)
%         k_tmp(6) = 0;
%         k_tmp(4) = k_tmp(3) * 0.8;
%     end
    if fb_id_out == id
        for i = 1:6
            if fb_q(i) < abs(k_tmp(i))
                temp1(i) = fb_u(i) + k_tmp(i) / ns;
                temp2(i) = fb_q(i) + abs(k_tmp(i) / ns);              
            else
                temp1(i) = fb_u(i);
            end
        end
    else
        for i = 1:6
            temp2(i) = 0;
        end
    end

% pause(ts*0.05);
u = temp1;
q = temp2;
id_out = id;
